simulink model "my_quadrotor_disturbance"  (R2017b)
settings: Solver=VariableStepAuto  StartTime=0.0  StopTime=10.0  RelTol=1e-3
libraries: simulink x4
settings Model: Creator=apple  LastModifiedBy=apple

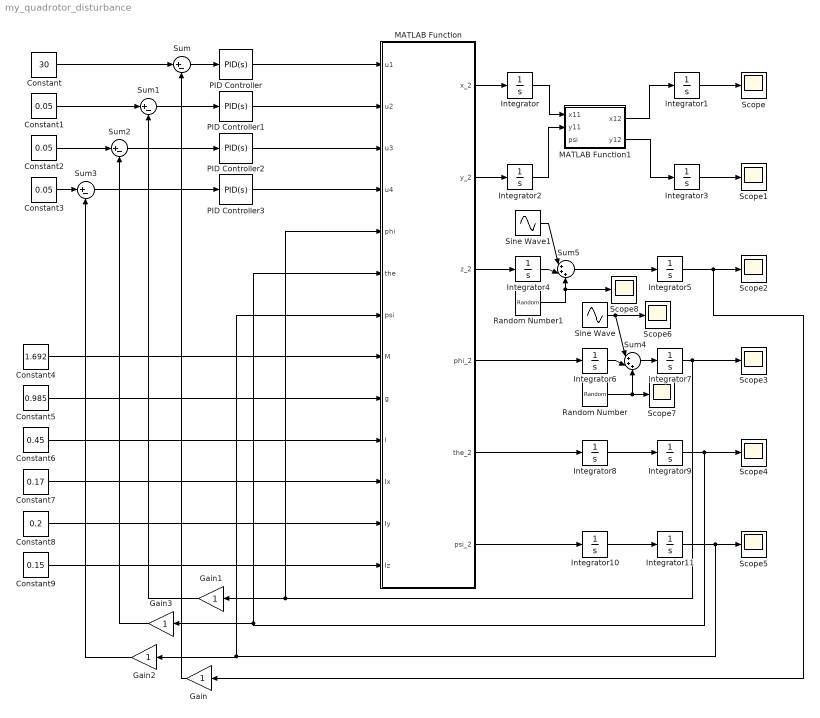
== system my_quadrotor_disturbance ==
  Constant : Constant  Value=30
  Constant1 : Constant  Value=0.05
  Constant2 : Constant  Value=0.05
  Constant3 : Constant  Value=0.05
  Constant4 : Constant  Value=1.692
  Constant5 : Constant  Value=0.985
  Constant6 : Constant  Value=0.45
  Constant7 : Constant  Value=0.17
  Constant8 : Constant  Value=0.2
  Constant9 : Constant  Value=0.15
  Gain{,1..3} (4 alike) : Gain
  Integrator{,1..11} (12 alike) : Integrator
  MATLAB Function : MATLAB Function  TreatAsAtomicUnit=on
  MATLAB Function1 : MATLAB Function  TreatAsAtomicUnit=on
  PID Controller{,1..3} (4 alike) : simulink/Continuous/PID Controller  Controller=PID  TimeDomain=Continuous-time  SampleTime=-1  IntegratorMethod=Forward Euler  FilterMethod=Forward Euler  Form=Parallel  UseFilter=on  ControllerParametersSource=internal  P=10  I=0.1  D=5  N=100  InitialConditionSource=internal  InitialConditionForIntegrator=0  InitialConditionForFilter=0  ExternalReset=none  LimitOutput=off  UpperSaturationLimit=inf  LowerSaturationLimit=-inf  LinearizeAsGain=on  AntiWindupMode=none  Kb=1  TrackingMode=off  Kt=1  PParamMin=[]  PParamMax=[]  IParamMin=[]  IParamMax=[]  DParamMin=[]  DParamMax=[]  NParamMin=[]  NParamMax=[]  KbParamMin=[]  KbParamMax=[]  KtParamMin=[]  KtParamMax=[]  POutMin=[]  POutMax=[]  IOutMin=[]  IOutMax=[]  DOutMin=[]  DOutMax=[]  NOutMin=[]  NOutMax=[]  KbOutMin=[]  KbOutMax=[]  KtOutMin=[]  KtOutMax=[]  IntegratorOutMin=[]  IntegratorOutMax=[]  FilterOutMin=[]  FilterOutMax=[]  SumOutMin=[]  SumOutMax=[]  SumI1OutMin=[]  SumI1OutMax=[]  SumI2OutMin=[]  SumI2OutMax=[]  SumI3OutMin=[]  SumI3OutMax=[]  SumDOutMin=[]  SumDOutMax=[]  SaturationOutMin=[]  SaturationOutMax=[]  IntegratorContinuousStateAttributes=''  IntegratorStateMustResolveToSignalObject=off  IntegratorRTWStateStorageClass=Auto  FilterContinuousStateAttributes=''  FilterStateMustResolveToSignalObject=off  FilterRTWStateStorageClass=Auto  DifferentiatorICPrevScaledInput=0  DifferentiatorOutMin=[]  DifferentiatorOutMax=[]  InitialConditionSetting=State (most efficient)  FilterDiffOutCoefMin=[]  FilterDiffOutCoefMax=[]  SumDenOutMin=[]  SumDenOutMax=[]  SumNumOutMin=[]  SumNumOutMax=[]  ReciprocalOutMin=[]  ReciprocalOutMax=[]  DivideOutMin=[]  DivideOutMax=[]  TunerSelectOption=Transfer Function Based (PID Tuner App)
  Random Number : RandomNumber  Variance=0.2  SampleTime=0.1
  Random Number1 : RandomNumber  Variance=20  SampleTime=0.01
  Scope{,1..8} (9 alike) : Scope
  Sine Wave : Sin  Amplitude=0.2  Frequency=3  SampleTime=0
  Sine Wave1 : Sin  Amplitude=5  Frequency=10  SampleTime=0
  Sum{,1..3} (4 alike) : Sum  Inputs=|+-
  Sum4 : Sum  Inputs=|+++
  Sum5 : Sum  Inputs=|+++
  wires:
  Constant/1 -> Sum/1
  Constant1/1 -> Sum1/1
  Constant2/1 -> Sum2/1
  Constant3/1 -> Sum3/1
  Integrator5/1 -> Gain/1, Scope2/1
  Integrator7/1 -> Scope3/1, Gain1/1, MATLAB Function/5(phi)
  MATLAB Function/4(phi_2) -> Integrator6/1
  Integrator8/1 -> Integrator9/1
  Integrator9/1 -> MATLAB Function/6(the), Gain3/1, Scope4/1
  MATLAB Function/5(the_2) -> Integrator8/1
  Integrator10/1 -> Integrator11/1
  Integrator11/1 -> Gain2/1, MATLAB Function/7(psi), Scope5/1
  MATLAB Function/6(psi_2) -> Integrator10/1
  Sum/1 -> PID Controller/1
  PID Controller/1 -> MATLAB Function/1(u1)
  Sum1/1 -> PID Controller1/1
  PID Controller1/1 -> MATLAB Function/2(u2)
  Sum2/1 -> PID Controller2/1
  Sum3/1 -> PID Controller3/1
  PID Controller2/1 -> MATLAB Function/3(u3)
  PID Controller3/1 -> MATLAB Function/4(u4)
  Gain/1 -> Sum/2
  Gain1/1 -> Sum1/2
  Gain3/1 -> Sum2/2
  Gain2/1 -> Sum3/2
  Constant4/1 -> MATLAB Function/8(M)
  Constant5/1 -> MATLAB Function/9(g)
  Constant6/1 -> MATLAB Function/10(l)
  Constant7/1 -> MATLAB Function/11(Ix)
  Constant8/1 -> MATLAB Function/12(Iy)
  Constant9/1 -> MATLAB Function/13(Iz)
  Integrator2/1 -> MATLAB Function1/2(y11)
  Integrator/1 -> MATLAB Function1/1(x11)
  MATLAB Function1/1(x12) -> Integrator1/1
  MATLAB Function1/2(y12) -> Integrator3/1
  MATLAB Function/1(x_2) -> Integrator/1
  MATLAB Function/2(y_2) -> Integrator2/1
  Integrator1/1 -> Scope/1
  Integrator3/1 -> Scope1/1
  Sum4/1 -> Integrator7/1
  Sine Wave/1 -> Scope6/1, Sum4/1
  Integrator6/1 -> Sum4/2
  Random Number/1 -> Scope7/1, Sum4/3
  Random Number1/1 -> Scope8/1, Sum5/3
  Sum5/1 -> Integrator5/1
  Sine Wave1/1 -> Sum5/1
  Integrator4/1 -> Sum5/2
  MATLAB Function/3(z_2) -> Integrator4/1

== matlab function my_quadrotor_disturbance/MATLAB Function ==
  data: u1 input; x_2 output; u2 input; u3 input; u4 input; phi input; the input; psi input; M input; g input; l input; Ix input; Iy input; Iz input; y_2 output; z_2 output; phi_2 output; the_2 output; psi_2 output
function [x_2, y_2, z_2, phi_2, the_2, psi_2] = dynamics(u1,u2,u3,u4,phi,the,psi,M,g,l,Ix,Iy,Iz)
x_2 = u1*(cos(phi)*sin(the)*cos(psi)+sin(phi)*sin(psi))/M;
y_2 = u1*(cos(phi)*sin(the)*cos(psi)-sin(phi)*sin(psi))/M;
z_2 = -g+u1*(cos(the)*cos(phi))/M;
phi_2 = l*u2/Ix;
the_2 = l*u3/Iy;
psi_2 = l*u4/Iz;

== matlab function my_quadrotor_disturbance/MATLAB Function1 ==
  data: x11 input; x12 output; y11 input; psi input; y12 output
function [x12,y12] = rot(x11,y11,psi)

x12 = x11 * cos(psi) - y11 * sin(psi);
y12 = x11 * sin(psi) + y11 * cos(psi);
